simulink model "Boeing787_OldMission_ElectricalThermalHydraulicFuelECS"  (R2013a)
settings: Solver=ode23tb  SolverMode=SingleTasking  StartTime=0.0  StopTime=346  RelTol=1e-3
InitFcn:
  | load('SampleOutput.mat')
  | 
  | load('SampleFuelBurn.mat')
undefined symbols (not defined in the file or in its folder): ailerons, AirProp, B_737, elevator, FuelBurn, HydProp, landing_gear, rudder, thrust_rev
libraries: PowerFlowLib x118, simulink x20
(part 24 of 26)

== system Boeing787_OldMission_ElectricalThermalHydraulicFuelECS/ECS/Right Pack1/Primary HX (air-air)/Thermal_resistance_KpW_cold ==
  Convective_HTC : Inport
  HX_parameters : Inport  Port=2
  Fin_parameters : Inport  Port=3
  Add : Sum
  Bus Selector : BusSelector  OutputSignals=N_f
  Bus Selector1 : BusSelector  OutputSignals=s_fin,l_fin,eta_fin,h_fin
  Calc_R_tot : Product  Inputs=**
  Calc_R_tot1 : Product  Inputs=*/
  Constant : Constant  Value=2
  Gain : Gain  Gain=2
  R1_Convection_to_plate/fin_base : Product  Inputs=////
  R1_convection_fin_or_plate_base_KpW : Display
  R5_Conv-conduction_through fin_projection : Product  Inputs=//////
  R5_convection_fin_projection_KpW : Display
  R_tot_K/W : Outport
  wires:
  HX_parameters/1 -> Bus Selector/1
  Fin_parameters/1 -> Bus Selector1/1
  Convective_HTC/1 -> R1_Convection_to_plate/fin_base/1, R5_Conv-conduction_through fin_projection/3  "HTC_Wpm2K"
  Bus Selector/1 -> R1_Convection_to_plate/fin_base/2, R5_Conv-conduction_through fin_projection/4  "<N_f>"
  Bus Selector1/1 -> R1_Convection_to_plate/fin_base/3  "<s_fin>"
  Bus Selector1/2 -> R1_Convection_to_plate/fin_base/4, R5_Conv-conduction_through fin_projection/6  "<l_fin>"
  R1_Convection_to_plate/fin_base/1 -> R1_convection_fin_or_plate_base_KpW/1, Calc_R_tot/1, Add/1
  Constant/1 -> R5_Conv-conduction_through fin_projection/1
  Bus Selector1/3 -> R5_Conv-conduction_through fin_projection/2  "<eta_fin>"
  Bus Selector1/4 -> R5_Conv-conduction_through fin_projection/5  "<h_fin>"
  R5_Conv-conduction_through fin_projection/1 -> R5_convection_fin_projection_KpW/1, Calc_R_tot/2, Gain/1
  Gain/1 -> Add/2
  Calc_R_tot/1 -> Calc_R_tot1/1  "R1R5"
  Add/1 -> Calc_R_tot1/2  "R1+2R5"
  Calc_R_tot1/1 -> R_tot_K/W/1  "Rtot"

== system Boeing787_OldMission_ElectricalThermalHydraulicFuelECS/ECS/Right Pack1/Primary HX (air-air)/Thermal_resistance_KpW_hot ==
  Convective_HTC : Inport
  HX_parameters : Inport  Port=2
  Fin_parameters : Inport  Port=3
  Add : Sum
  Bus Selector : BusSelector  OutputSignals=N_f
  Bus Selector1 : BusSelector  OutputSignals=s_fin,l_fin,eta_fin,h_fin
  Calc_R_tot : Product  Inputs=**
  Calc_R_tot1 : Product  Inputs=*/
  Constant : Constant  Value=2
  Gain : Gain  Gain=2
  R1_Convection_to_plate/fin_base : Product  Inputs=////
  R1_convection_fin_or_plate_base_KpW : Display
  R5_Conv-conduction_through fin_projection : Product  Inputs=//////
  R5_convection_fin_projection_KpW : Display
  R_tot_K/W : Outport
  wires:
  Calc_R_tot1/1 -> R_tot_K/W/1  "Rtot"
  Add/1 -> Calc_R_tot1/2  "R1+2R5"
  Calc_R_tot/1 -> Calc_R_tot1/1  "R1R5"
  Gain/1 -> Add/2
  R5_Conv-conduction_through fin_projection/1 -> Gain/1, Calc_R_tot/2, R5_convection_fin_projection_KpW/1
  Bus Selector1/4 -> R5_Conv-conduction_through fin_projection/5  "<h_fin>"
  Bus Selector1/3 -> R5_Conv-conduction_through fin_projection/2  "<eta_fin>"
  Constant/1 -> R5_Conv-conduction_through fin_projection/1
  R1_Convection_to_plate/fin_base/1 -> Add/1, Calc_R_tot/1, R1_convection_fin_or_plate_base_KpW/1
  Bus Selector1/2 -> R5_Conv-conduction_through fin_projection/6, R1_Convection_to_plate/fin_base/4  "<l_fin>"
  Bus Selector1/1 -> R1_Convection_to_plate/fin_base/3  "<s_fin>"
  Bus Selector/1 -> R5_Conv-conduction_through fin_projection/4, R1_Convection_to_plate/fin_base/2  "<N_f>"
  Convective_HTC/1 -> R5_Conv-conduction_through fin_projection/3, R1_Convection_to_plate/fin_base/1  "HTC_Wpm2K"
  Fin_parameters/1 -> Bus Selector1/1
  HX_parameters/1 -> Bus Selector/1

== system Boeing787_OldMission_ElectricalThermalHydraulicFuelECS/ECS/Right Pack1/Primary HX (air-air)/convective_HTC_Wm-2K-1_cold ==
  Colburn_J_factor : Inport
  Re : Inport  Port=2
  air_properties : Inport  Port=3
  hydraulic_diameter : Inport  Port=4
  Bus Selector : BusSelector  OutputSignals=Pr,K_air
  Constant : Constant  Value=1/3
  Divide : Product  Inputs=****/
  Math Function : Math  Operator=pow  SaturateOnIntegerOverflow=on
  Convective_HTC_Wm-2K-1 : Outport
  wires:
  air_properties/1 -> Bus Selector/1
  Colburn_J_factor/1 -> Divide/1
  Re/1 -> Divide/2
  Bus Selector/1 -> Math Function/1  "<Pr>"
  Constant/1 -> Math Function/2
  Math Function/1 -> Divide/3
  Bus Selector/2 -> Divide/4  "<K_air>"
  hydraulic_diameter/1 -> Divide/5
  Divide/1 -> Convective_HTC_Wm-2K-1/1

== system Boeing787_OldMission_ElectricalThermalHydraulicFuelECS/ECS/Right Pack1/Primary HX (air-air)/convective_HTC_Wm-2K-1_hot ==
  Colburn_J_factor : Inport
  Re : Inport  Port=2
  air_properties : Inport  Port=3
  hydraulic_diameter : Inport  Port=4
  Bus Selector : BusSelector  OutputSignals=Pr,K_air
  Constant : Constant  Value=1/3
  Divide : Product  Inputs=****/
  Math Function : Math  Operator=pow  SaturateOnIntegerOverflow=on
  Convective_HTC_Wm-2K-1 : Outport
  wires:
  Divide/1 -> Convective_HTC_Wm-2K-1/1
  hydraulic_diameter/1 -> Divide/5
  Bus Selector/2 -> Divide/4  "<K_air>"
  Math Function/1 -> Divide/3
  Constant/1 -> Math Function/2
  Bus Selector/1 -> Math Function/1  "<Pr>"
  Re/1 -> Divide/2
  Colburn_J_factor/1 -> Divide/1
  air_properties/1 -> Bus Selector/1

== system Boeing787_OldMission_ElectricalThermalHydraulicFuelECS/ECS/Right Pack1/Secondary HX (air-air)1/Air_properties_in_flows_hot_and_cold ==
  In_flow_bus_hot : Inport
  In_flow_bus_cold : Inport  Port=2
  Bus Creator : BusCreator  Inputs=5
  Bus Creator3 : BusCreator  Inputs=5
  air_properties_in_cold : Subsystem
  air_properties_in_hot : Subsystem
  air_properties_in_hot1 : Outport
  air_properties_in_cold1 : Outport  Port=2
  wires:
  air_properties_in_hot/4(K_air_Wm-1K-2) -> Bus Creator/4  "K_air"
  air_properties_in_cold/5(Pr) -> Bus Creator3/5  "Pr"
  air_properties_in_hot/5(Pr) -> Bus Creator/5  "Pr"
  In_flow_bus_cold/1 -> air_properties_in_cold/1(In_flow_bus_cold)
  In_flow_bus_hot/1 -> air_properties_in_hot/1(In_flow_bus_hot)
  Bus Creator/1 -> air_properties_in_hot1/1
  Bus Creator3/1 -> air_properties_in_cold1/1
  air_properties_in_hot/3(mu_air_Pa.s) -> Bus Creator/3  "mu_air"
  air_properties_in_hot/2(cp_air_Jkg-1K-1) -> Bus Creator/2  "cp_air"
  air_properties_in_hot/1(rho_air_kgm-3) -> Bus Creator/1  "rho_air"
  air_properties_in_cold/4(K_air_Wm-1K-2) -> Bus Creator3/4  "K_air"
  air_properties_in_cold/3(mu_air_Pa.s) -> Bus Creator3/3  "mu_air"
  air_properties_in_cold/2(cp_air_Jkg-1K-1) -> Bus Creator3/2  "cp_air"
  air_properties_in_cold/1(rho_air_kgm-3) -> Bus Creator3/1  "rho_air"

== system Boeing787_OldMission_ElectricalThermalHydraulicFuelECS/ECS/Right Pack1/Secondary HX (air-air)1/C_T_c_av ==
  In_flow_bus : Inport
  air_properties : Inport  Port=2
  Tot_thermal_resist : Inport  Port=3
  Add : Sum
  Bus Selector : BusSelector  OutputSignals=mdot_kgps
  Bus Selector1 : BusSelector  OutputSignals=cp_air
  Constant : Constant
  Divide : Product  Inputs=***
  Divide1 : Product  Inputs=*/
  Gain : Gain  Gain=2
  C_T_c_av : Outport
  wires:
  Divide1/1 -> C_T_c_av/1
  Add/1 -> Divide1/2
  Constant/1 -> Add/2
  Gain/1 -> Divide1/1, Add/1
  Divide/1 -> Gain/1
  Bus Selector1/1 -> Divide/3  "<cp_air>"
  Bus Selector/1 -> Divide/2  "<mdot_kgps>"
  Tot_thermal_resist/1 -> Divide/1  "R_tot_c"
  In_flow_bus/1 -> Bus Selector/1
  air_properties/1 -> Bus Selector1/1

== system Boeing787_OldMission_ElectricalThermalHydraulicFuelECS/ECS/Right Pack1/Secondary HX (air-air)1/C_T_c_i ==
  In_flow_bus : Inport
  air_properties : Inport  Port=2
  Tot_thermal_resist : Inport  Port=3
  HX_parameters : Inport  Port=4
  Add : Sum
  Bus Selector : BusSelector  OutputSignals=mdot_kgps
  Bus Selector1 : BusSelector  OutputSignals=cp_air
  Bus Selector2 : BusSelector  OutputSignals=m_cm,cp_hx
  Constant : Constant
  Divide : Product  Inputs=***
  Divide2 : Product  Inputs=**///
  Gain : Gain  Gain=2
  Gain1 : Gain  Gain=2
  C_T_c_i : Outport
  wires:
  In_flow_bus/1 -> Bus Selector/1
  air_properties/1 -> Bus Selector1/1
  Tot_thermal_resist/1 -> Divide/1  "R_tot"
  Bus Selector/1 -> Divide/2, Divide2/1  "<mdot_kgps>"
  Bus Selector1/1 -> Divide/3, Divide2/2  "<cp_air>"
  Divide/1 -> Gain/1
  Gain/1 -> Add/1
  Constant/1 -> Add/2
  HX_parameters/1 -> Bus Selector2/1
  Bus Selector2/1 -> Divide2/3  "<m_cm>"
  Bus Selector2/2 -> Divide2/4  "<cp_hx>"
  Add/1 -> Divide2/5
  Gain1/1 -> C_T_c_i/1
  Divide2/1 -> Gain1/1

== system Boeing787_OldMission_ElectricalThermalHydraulicFuelECS/ECS/Right Pack1/Secondary HX (air-air)1/C_T_h_av ==
  In_flow_bus : Inport
  air_properties : Inport  Port=2
  Tot_thermal_resist : Inport  Port=3
  Add : Sum
  Bus Selector : BusSelector  OutputSignals=mdot_kgps
  Bus Selector1 : BusSelector  OutputSignals=cp_air
  Constant : Constant
  Divide : Product  Inputs=***
  Divide1 : Product  Inputs=*/
  Gain : Gain  Gain=2
  C_T_h_av : Outport
  wires:
  Divide1/1 -> C_T_h_av/1
  Add/1 -> Divide1/2
  Constant/1 -> Add/2
  Gain/1 -> Divide1/1, Add/1
  Divide/1 -> Gain/1
  Bus Selector1/1 -> Divide/3  "<cp_air>"
  Bus Selector/1 -> Divide/2  "<mdot_kgps>"
  Tot_thermal_resist/1 -> Divide/1  "R_tot_h"
  In_flow_bus/1 -> Bus Selector/1
  air_properties/1 -> Bus Selector1/1

== system Boeing787_OldMission_ElectricalThermalHydraulicFuelECS/ECS/Right Pack1/Secondary HX (air-air)1/C_T_h_i ==
  In_flow_bus : Inport
  air_properties : Inport  Port=2
  Tot_thermal_resist : Inport  Port=3
  HX_parameters : Inport  Port=4
  Add : Sum
  Bus Selector : BusSelector  OutputSignals=mdot_kgps
  Bus Selector1 : BusSelector  OutputSignals=cp_air
  Bus Selector2 : BusSelector  OutputSignals=m_cm,cp_hx
  Constant : Constant
  Divide : Product  Inputs=***
  Divide2 : Product  Inputs=**///
  Gain : Gain  Gain=2
  Gain1 : Gain  Gain=2
  C_T_h_i : Outport
  wires:
  Gain1/1 -> C_T_h_i/1
  Add/1 -> Divide2/5
  Bus Selector2/2 -> Divide2/4  "<cp_hx>"
  Bus Selector2/1 -> Divide2/3  "<m_cm>"
  HX_parameters/1 -> Bus Selector2/1
  Constant/1 -> Add/2
  Gain/1 -> Add/1
  Divide/1 -> Gain/1
  Bus Selector1/1 -> Divide/3, Divide2/2  "<cp_air>"
  Bus Selector/1 -> Divide/2, Divide2/1  "<mdot_kgps>"
  Tot_thermal_resist/1 -> Divide/1  "R_tot_h"
  air_properties/1 -> Bus Selector1/1
  In_flow_bus/1 -> Bus Selector/1
  Divide2/1 -> Gain1/1

== system Boeing787_OldMission_ElectricalThermalHydraulicFuelECS/ECS/Right Pack1/Secondary HX (air-air)1/Calculating_T_c_av ==
  T_cm : Inport
  In_flow_bus : Inport  Port=2
  C_t_c_av : Inport  Port=3
  Add1 : Sum  Inputs=-+
  Add3 : Sum
  Bus Selector : BusSelector  OutputSignals=temp_C
  Divide1 : Product  Inputs=**
  T_c_av_degreC : Outport
  wires:
  T_cm/1 -> Add3/1, Add1/1  "T_cm"
  In_flow_bus/1 -> Bus Selector/1
  Bus Selector/1 -> Add1/2  "<temp_C>"
  C_t_c_av/1 -> Divide1/2
  Add1/1 -> Divide1/1  "T_c_i - T_cm"
  Divide1/1 -> Add3/2
  Add3/1 -> T_c_av_degreC/1

== system Boeing787_OldMission_ElectricalThermalHydraulicFuelECS/ECS/Right Pack1/Secondary HX (air-air)1/Calculating_T_h_av ==
  T_cm : Inport
  In_flow_bus : Inport  Port=2
  C_t_h_av : Inport  Port=3
  Add1 : Sum  Inputs=-+
  Add3 : Sum
  Bus Selector : BusSelector  OutputSignals=temp_C
  Divide1 : Product  Inputs=**
  T_h_av_degreC : Outport
  wires:
  Add1/1 -> Divide1/1  "T_h_i - T_cm"
  C_t_h_av/1 -> Divide1/2
  Bus Selector/1 -> Add1/2  "<temp_C>"
  In_flow_bus/1 -> Bus Selector/1
  T_cm/1 -> Add1/1, Add3/1  "T_cm"
  Add3/1 -> T_h_av_degreC/1
  Divide1/1 -> Add3/2

== system Boeing787_OldMission_ElectricalThermalHydraulicFuelECS/ECS/Right Pack1/Secondary HX (air-air)1/Calculating_core_mass_temp ==
  note: dTcm/dt
  note: Tcm
  C_T_h_i : Inport
  C_T_c_i : Inport  Port=2
  C_t_cm : Inport  Port=3
  In_flow_bus_hot : Inport  Port=4
  In_flow_bus_cold : Inport  Port=5
  Add : Sum  Inputs=++-
  Bus Selector : BusSelector  OutputSignals=temp_C
  Bus Selector1 : BusSelector  OutputSignals=temp_C
  Divide : Product  Inputs=**
  Divide1 : Product  Inputs=**
  Divide2 : Product  Inputs=**
  Integrator : Integrator  InitialCondition=T_cm_0
  Core_mass_temp_C : Outport
  wires:
  Divide1/1 -> Add/3
  C_t_cm/1 -> Divide1/2
  Integrator/1 -> Core_mass_temp_C/1, Divide1/1
  Add/1 -> Integrator/1
  Divide2/1 -> Add/2
  Divide/1 -> Add/1
  Bus Selector1/1 -> Divide2/2  "<temp_C>"
  C_T_c_i/1 -> Divide2/1
  Bus Selector/1 -> Divide/2  "<temp_C>"
  C_T_h_i/1 -> Divide/1
  In_flow_bus_cold/1 -> Bus Selector1/1
  In_flow_bus_hot/1 -> Bus Selector/1

== system Boeing787_OldMission_ElectricalThermalHydraulicFuelECS/ECS/Right Pack1/Secondary HX (air-air)1/Colburn_J_factor_cold ==
  Fin_prameter_ratios : Inport
  Re : Inport  Port=2
  Add : Sum
  Bus Selector : BusSelector  OutputSignals=alpha_fin,delta_fin,gamma_fin
  Constant : Constant  Value=-0.5403
  Constant1 : Constant  Value=-0.1541
  Constant2 : Constant  Value=0.1499
  Constant3 : Constant  Value=-0.0678
  Constant4 : Constant  Value=1.34
  Constant5 : Constant  Value=0.504
  Constant6 : Constant  Value=0.456
  Constant7 : Constant  Value=-1.055
  Constant8 : Constant
  Constant9 : Constant  Value=0.1
  Divide : Product  Inputs=****
  Divide1 : Product  Inputs=****
  Divide2 : Product  Inputs=**
  Gain : Gain  Gain=0.6522
  Gain1 : Gain  Gain=5.269*10^(-5)
  Re1 : Math  Operator=pow  SaturateOnIntegerOverflow=on
  Re2 : Math  Operator=pow  SaturateOnIntegerOverflow=on
  alpha_fin : Math  Operator=pow  SaturateOnIntegerOverflow=on
  alpha_fin1 : Math  Operator=pow  SaturateOnIntegerOverflow=on
  delta_fin : Math  Operator=pow  SaturateOnIntegerOverflow=on
  delta_fin1 : Math  Operator=pow  SaturateOnIntegerOverflow=on
  gamma_fin : Math  Operator=pow  SaturateOnIntegerOverflow=on
  gamma_fin1 : Math  Operator=pow  SaturateOnIntegerOverflow=on
  gamma_fin2 : Math  Operator=pow  SaturateOnIntegerOverflow=on
  Colburn_J_factor : Outport
  wires:
  Divide2/1 -> Colburn_J_factor/1
  Gain/1 -> Divide2/1
  gamma_fin2/1 -> Divide2/2
  Constant9/1 -> gamma_fin2/2
  Add/1 -> gamma_fin2/1
  Gain1/1 -> Add/1
  Constant8/1 -> Add/2
  Divide1/1 -> Gain1/1
  gamma_fin1/1 -> Divide1/4
  delta_fin1/1 -> Divide1/3
  alpha_fin1/1 -> Divide1/2
  Re2/1 -> Divide1/1
  Divide/1 -> Gain/1
  gamma_fin/1 -> Divide/4
  delta_fin/1 -> Divide/3
  alpha_fin/1 -> Divide/2
  Re1/1 -> Divide/1
  Bus Selector/3 -> gamma_fin1/1, gamma_fin/1  "<gamma_fin>"
  Bus Selector/2 -> delta_fin1/1, delta_fin/1  "<delta_fin>"
  Bus Selector/1 -> alpha_fin1/1, alpha_fin/1  "<alpha_fin>"
  Re/1 -> Re2/1, Re1/1
  Constant7/1 -> gamma_fin1/2
  Constant6/1 -> delta_fin1/2
  Constant5/1 -> alpha_fin1/2
  Constant4/1 -> Re2/2
  Constant3/1 -> gamma_fin/2
  Constant2/1 -> delta_fin/2
  Constant1/1 -> alpha_fin/2
  Constant/1 -> Re1/2
  Fin_prameter_ratios/1 -> Bus Selector/1

== system Boeing787_OldMission_ElectricalThermalHydraulicFuelECS/ECS/Right Pack1/Secondary HX (air-air)1/Colburn_J_factor_hot ==
  Fin_prameter_ratios : Inport
  Re : Inport  Port=2
  Add : Sum
  Bus Selector : BusSelector  OutputSignals=alpha_fin,delta_fin,gamma_fin
  Constant : Constant  Value=-0.5403
  Constant1 : Constant  Value=-0.1541
  Constant2 : Constant  Value=0.1499
  Constant3 : Constant  Value=-0.0678
  Constant4 : Constant  Value=1.34
  Constant5 : Constant  Value=0.504
  Constant6 : Constant  Value=0.456
  Constant7 : Constant  Value=-1.055
  Constant8 : Constant
  Constant9 : Constant  Value=0.1
  Divide : Product  Inputs=****
  Divide1 : Product  Inputs=****
  Divide2 : Product  Inputs=**
  Gain : Gain  Gain=0.6522
  Gain1 : Gain  Gain=5.269*10^(-5)
  Re1 : Math  Operator=pow  SaturateOnIntegerOverflow=on
  Re2 : Math  Operator=pow  SaturateOnIntegerOverflow=on
  alpha_fin : Math  Operator=pow  SaturateOnIntegerOverflow=on
  alpha_fin1 : Math  Operator=pow  SaturateOnIntegerOverflow=on
  delta_fin : Math  Operator=pow  SaturateOnIntegerOverflow=on
  delta_fin1 : Math  Operator=pow  SaturateOnIntegerOverflow=on
  gamma_fin : Math  Operator=pow  SaturateOnIntegerOverflow=on
  gamma_fin1 : Math  Operator=pow  SaturateOnIntegerOverflow=on
  gamma_fin2 : Math  Operator=pow  SaturateOnIntegerOverflow=on
  Colburn_J_factor : Outport
  wires:
  Fin_prameter_ratios/1 -> Bus Selector/1
  Constant/1 -> Re1/2
  Constant1/1 -> alpha_fin/2
  Constant2/1 -> delta_fin/2
  Constant3/1 -> gamma_fin/2
  Constant4/1 -> Re2/2
  Constant5/1 -> alpha_fin1/2
  Constant6/1 -> delta_fin1/2
  Constant7/1 -> gamma_fin1/2
  Re/1 -> Re1/1, Re2/1
  Bus Selector/1 -> alpha_fin/1, alpha_fin1/1  "<alpha_fin>"
  Bus Selector/2 -> delta_fin/1, delta_fin1/1  "<delta_fin>"
  Bus Selector/3 -> gamma_fin/1, gamma_fin1/1  "<gamma_fin>"
  Re1/1 -> Divide/1
  alpha_fin/1 -> Divide/2
  delta_fin/1 -> Divide/3
  gamma_fin/1 -> Divide/4
  Divide/1 -> Gain/1
  Re2/1 -> Divide1/1
  alpha_fin1/1 -> Divide1/2
  delta_fin1/1 -> Divide1/3
  gamma_fin1/1 -> Divide1/4
  Divide1/1 -> Gain1/1
  Constant8/1 -> Add/2
  Gain1/1 -> Add/1
  Add/1 -> gamma_fin2/1
  Constant9/1 -> gamma_fin2/2
  gamma_fin2/1 -> Divide2/2
  Gain/1 -> Divide2/1
  Divide2/1 -> Colburn_J_factor/1

== system Boeing787_OldMission_ElectricalThermalHydraulicFuelECS/ECS/Right Pack1/Secondary HX (air-air)1/Friction_factor_cold ==
  Fin_prameter_ratios : Inport
  Re : Inport  Port=2
  Add : Sum
  Bus Selector : BusSelector  OutputSignals=alpha_fin,delta_fin,gamma_fin
  Constant : Constant  Value=-0.7422
  Constant1 : Constant  Value=-0.1856
  Constant2 : Constant  Value=0.3053
  Constant3 : Constant  Value=-0.2659
  Constant4 : Constant  Value=4.429
  Constant5 : Constant  Value=0.92
  Constant6 : Constant  Value=3.767
  Constant7 : Constant  Value=0.236
  Constant8 : Constant
  Constant9 : Constant  Value=0.1
  Divide : Product  Inputs=****
  Divide1 : Product  Inputs=****
  Divide2 : Product  Inputs=**
  Gain : Gain  Gain=9.6243
  Gain1 : Gain  Gain=7.669*10^(-8)
  Re1 : Math  Operator=pow  SaturateOnIntegerOverflow=on
  Re2 : Math  Operator=pow  SaturateOnIntegerOverflow=on
  alpha_fin : Math  Operator=pow  SaturateOnIntegerOverflow=on
  alpha_fin1 : Math  Operator=pow  SaturateOnIntegerOverflow=on
  delta_fin : Math  Operator=pow  SaturateOnIntegerOverflow=on
  delta_fin1 : Math  Operator=pow  SaturateOnIntegerOverflow=on
  gamma_fin : Math  Operator=pow  SaturateOnIntegerOverflow=on
  gamma_fin1 : Math  Operator=pow  SaturateOnIntegerOverflow=on
  gamma_fin2 : Math  Operator=pow  SaturateOnIntegerOverflow=on
  Friction_factor : Outport
  wires:
  Fin_prameter_ratios/1 -> Bus Selector/1
  Constant/1 -> Re1/2
  Constant1/1 -> alpha_fin/2
  Constant2/1 -> delta_fin/2
  Constant3/1 -> gamma_fin/2
  Constant4/1 -> Re2/2
  Constant5/1 -> alpha_fin1/2
  Constant6/1 -> delta_fin1/2
  Constant7/1 -> gamma_fin1/2
  Re/1 -> Re1/1, Re2/1
  Bus Selector/1 -> alpha_fin/1, alpha_fin1/1  "<alpha_fin>"
  Bus Selector/2 -> delta_fin/1, delta_fin1/1  "<delta_fin>"
  Bus Selector/3 -> gamma_fin/1, gamma_fin1/1  "<gamma_fin>"
  Re1/1 -> Divide/1
  alpha_fin/1 -> Divide/2
  delta_fin/1 -> Divide/3
  gamma_fin/1 -> Divide/4
  Divide/1 -> Gain/1
  Re2/1 -> Divide1/1
  alpha_fin1/1 -> Divide1/2
  delta_fin1/1 -> Divide1/3
  gamma_fin1/1 -> Divide1/4
  Divide1/1 -> Gain1/1
  Constant8/1 -> Add/2
  Gain1/1 -> Add/1
  Add/1 -> gamma_fin2/1
  Constant9/1 -> gamma_fin2/2
  gamma_fin2/1 -> Divide2/2
  Gain/1 -> Divide2/1
  Divide2/1 -> Friction_factor/1

== system Boeing787_OldMission_ElectricalThermalHydraulicFuelECS/ECS/Right Pack1/Secondary HX (air-air)1/Friction_factor_hot ==
  Fin_prameter_ratios : Inport
  Re : Inport  Port=2
  Add : Sum
  Bus Selector : BusSelector  OutputSignals=alpha_fin,delta_fin,gamma_fin
  Constant : Constant  Value=-0.7422
  Constant1 : Constant  Value=-0.1856
  Constant2 : Constant  Value=0.3053
  Constant3 : Constant  Value=-0.2659
  Constant4 : Constant  Value=4.429
  Constant5 : Constant  Value=0.92
  Constant6 : Constant  Value=3.767
  Constant7 : Constant  Value=0.236
  Constant8 : Constant
  Constant9 : Constant  Value=0.1
  Divide : Product  Inputs=****
  Divide1 : Product  Inputs=****
  Divide2 : Product  Inputs=**
  Gain : Gain  Gain=9.6243
  Gain1 : Gain  Gain=7.669*10^(-8)
  Re1 : Math  Operator=pow  SaturateOnIntegerOverflow=on
  Re2 : Math  Operator=pow  SaturateOnIntegerOverflow=on
  alpha_fin : Math  Operator=pow  SaturateOnIntegerOverflow=on
  alpha_fin1 : Math  Operator=pow  SaturateOnIntegerOverflow=on
  delta_fin : Math  Operator=pow  SaturateOnIntegerOverflow=on
  delta_fin1 : Math  Operator=pow  SaturateOnIntegerOverflow=on
  gamma_fin : Math  Operator=pow  SaturateOnIntegerOverflow=on
  gamma_fin1 : Math  Operator=pow  SaturateOnIntegerOverflow=on
  gamma_fin2 : Math  Operator=pow  SaturateOnIntegerOverflow=on
  Friction_factor : Outport
  wires:
  Divide2/1 -> Friction_factor/1
  Gain/1 -> Divide2/1
  gamma_fin2/1 -> Divide2/2
  Constant9/1 -> gamma_fin2/2
  Add/1 -> gamma_fin2/1
  Gain1/1 -> Add/1
  Constant8/1 -> Add/2
  Divide1/1 -> Gain1/1
  gamma_fin1/1 -> Divide1/4
  delta_fin1/1 -> Divide1/3
  alpha_fin1/1 -> Divide1/2
  Re2/1 -> Divide1/1
  Divide/1 -> Gain/1
  gamma_fin/1 -> Divide/4
  delta_fin/1 -> Divide/3
  alpha_fin/1 -> Divide/2
  Re1/1 -> Divide/1
  Bus Selector/3 -> gamma_fin1/1, gamma_fin/1  "<gamma_fin>"
  Bus Selector/2 -> delta_fin1/1, delta_fin/1  "<delta_fin>"
  Bus Selector/1 -> alpha_fin1/1, alpha_fin/1  "<alpha_fin>"
  Re/1 -> Re2/1, Re1/1
  Constant7/1 -> gamma_fin1/2
  Constant6/1 -> delta_fin1/2
  Constant5/1 -> alpha_fin1/2
  Constant4/1 -> Re2/2
  Constant3/1 -> gamma_fin/2
  Constant2/1 -> delta_fin/2
  Constant1/1 -> alpha_fin/2
  Constant/1 -> Re1/2
  Fin_prameter_ratios/1 -> Bus Selector/1

== system Boeing787_OldMission_ElectricalThermalHydraulicFuelECS/ECS/Right Pack1/Secondary HX (air-air)1/HX_and_Fin_paramters ==
  Bus Creator1 : BusCreator  Inputs=6
  Bus Creator2 : BusCreator  Inputs=6
  Bus Creator3 : BusCreator  Inputs=3
  Fin_parameters : Subsystem
  HX_parameters : Subsystem
  Other_HX_parameters2 : Subsystem
  alpha : Product  Inputs=*/
  delta : Product  Inputs=*/
  gamma : Product  Inputs=*/
  HX_parameters2 : Outport
  Fin_parameters1 : Outport  Port=2
  Fin_parameters_ratios : Outport  Port=3
  wires:
  [Other_HX_parameters] -> HX_parameters/1(Other_HX_parameters)
  Other_HX_parameters2/1(Out1) -> [Other_HX_parameters]
  Bus Creator3/1 -> Fin_parameters_ratios/1
  gamma/1 -> Bus Creator3/3  "gamma_fin"
  delta/1 -> Bus Creator3/2  "delta_fin"
  alpha/1 -> Bus Creator3/1  "alpha_fin"
  Bus Creator1/1 -> HX_parameters2/1
  Bus Creator2/1 -> HX_parameters/2(Fin_parameters), Fin_parameters1/1
  HX_parameters/1(tot_free_flow_area_m^2) -> Bus Creator1/1  "A"
  Fin_parameters/3(Fin_free_flow_width_m) -> Bus Creator2/3, alpha/1, gamma/2  "s_fin"
  Fin_parameters/6(Fin_eff) -> Bus Creator2/6  "eta_fin"
  Fin_parameters/5(K_fin_Wm-1K-1) -> Bus Creator2/5  "K_n"
  Fin_parameters/4(Fin_free_flow_height_m) -> Bus Creator2/4, alpha/2  "h_fin"
  Fin_parameters/2(Fin_thickness_m) -> gamma/1, Bus Creator2/2, delta/1  "t_fin"
  Fin_parameters/1(Fin_length_m) -> Bus Creator2/1, delta/2  "l_fin"
  HX_parameters/6(m_hx_kg) -> Bus Creator1/6  "m_cm"
  HX_parameters/5(cp_hx_Jkg-1K-1) -> Bus Creator1/5  "cp_hx"
  HX_parameters/4(K_hx_Wm-1K-1) -> Bus Creator1/4  "K_p"
  HX_parameters/3(tot_no_of_fins_per_HX_per_flow) -> Bus Creator1/3  "N_f"
  HX_parameters/2(tot_length_in_direc_of_flow_m) -> Bus Creator1/2  "L_hx"

== system Boeing787_OldMission_ElectricalThermalHydraulicFuelECS/ECS/Right Pack1/Secondary HX (air-air)1/Heat_load_cold_side ==
  In_flow_bus : Inport
  air_properties : Inport  Port=2
  temp_out_degreeC : Inport  Port=3
  Bus Selector : BusSelector  OutputSignals=temp_C,mdot_kgps
  Bus Selector1 : BusSelector  OutputSignals=cp_air
  Product : Product  Inputs=3  RndMeth=Zero
  temp_diff : Sum  Inputs=-+
  Heat_rate_Watt : Outport
  wires:
  In_flow_bus/1 -> Bus Selector/1
  air_properties/1 -> Bus Selector1/1
  Bus Selector/1 -> temp_diff/1  "<temp_C>"
  temp_out_degreeC/1 -> temp_diff/2
  Bus Selector/2 -> Product/1  "<mdot_kgps>"
  Bus Selector1/1 -> Product/2  "<cp_air>"
  temp_diff/1 -> Product/3
  Product/1 -> Heat_rate_Watt/1

== system Boeing787_OldMission_ElectricalThermalHydraulicFuelECS/ECS/Right Pack1/Secondary HX (air-air)1/Heat_load_hot_side ==
  In_flow_bus : Inport
  air_properties : Inport  Port=2
  temp_out_degreeC : Inport  Port=3
  Bus Selector : BusSelector  OutputSignals=temp_C,mdot_kgps
  Bus Selector1 : BusSelector  OutputSignals=cp_air
  Product : Product  Inputs=3  RndMeth=Zero
  temp_diff : Sum  Inputs=+-
  Heat_rate_Watt : Outport
  wires:
  Product/1 -> Heat_rate_Watt/1
  temp_diff/1 -> Product/3
  Bus Selector1/1 -> Product/2  "<cp_air>"
  Bus Selector/2 -> Product/1  "<mdot_kgps>"
  temp_out_degreeC/1 -> temp_diff/2
  Bus Selector/1 -> temp_diff/1  "<temp_C>"
  air_properties/1 -> Bus Selector1/1
  In_flow_bus/1 -> Bus Selector/1

== system Boeing787_OldMission_ElectricalThermalHydraulicFuelECS/ECS/Right Pack1/Secondary HX (air-air)1/Hydraulic_diam_m ==
  Fin_parameters : Inport
  Add : Sum  Inputs=+++
  Add1 : Sum
  Bus Selector1 : BusSelector  OutputSignals=l_fin,t_fin,s_fin,h_fin,K_n,eta_fin
  Gain : Gain  Gain=4
  Gain1 : Gain  Gain=2
  Terminator : Terminator
  Terminator1 : Terminator
  hl : Product  Inputs=**
  shl : Product  Inputs=***
  sl : Product  Inputs=**
  th : Product  Inputs=**
  ts : Product  Inputs=**
  ts1 : Product  Inputs=*/
  Out1 : Outport
  wires:
  ts1/1 -> Out1/1
  Add1/1 -> ts1/2
  Gain/1 -> ts1/1
  ts/1 -> Add1/2
  Gain1/1 -> Add1/1
  Add/1 -> Gain1/1
  th/1 -> Add/3
  hl/1 -> Add/2
  sl/1 -> Add/1
  Bus Selector1/2 -> th/1, ts/1  "<t_fin>"
  shl/1 -> Gain/1
  Bus Selector1/1 -> hl/2, sl/2, shl/3  "<l_fin>"
  Bus Selector1/4 -> th/2, shl/2, hl/1  "<h_fin>"
  Bus Selector1/3 -> ts/2, sl/1, shl/1  "<s_fin>"
  Fin_parameters/1 -> Bus Selector1/1
  Bus Selector1/5 -> Terminator/1  "<K_n>"
  Bus Selector1/6 -> Terminator1/1  "<eta_fin>"

== system Boeing787_OldMission_ElectricalThermalHydraulicFuelECS/ECS/Right Pack1/Secondary HX (air-air)1/Pressure_drop_cold ==
  Friction_factor : Inport
  HX_parameters : Inport  Port=2
  air_properties : Inport  Port=3
  air_velocity : Inport  Port=4
  D_hydraulic : Inport  Port=5
  In_flow_bus : Inport  Port=6
  Add : Sum  Inputs=-+
  Bus Selector : BusSelector  OutputSignals=L_hx
  Bus Selector1 : BusSelector  OutputSignals=rho_air
  Bus Selector2 : BusSelector  OutputSignals=press_Pa
  Constant : Constant  Value=2
  Divide3 : Product  Inputs=****/
  Gain2 : Gain  Gain=2
  Math Function : Math  Operator=pow  SaturateOnIntegerOverflow=on
  pres_drop_Pa : Outport
  pres_Pa : Outport  Port=2
  wires:
  Friction_factor/1 -> Divide3/1
  HX_parameters/1 -> Bus Selector/1
  Bus Selector/1 -> Divide3/2  "<L_hx>"
  air_properties/1 -> Bus Selector1/1
  Bus Selector1/1 -> Divide3/3  "<rho_air>"
  air_velocity/1 -> Math Function/1
  Constant/1 -> Math Function/2
  Math Function/1 -> Divide3/4
  D_hydraulic/1 -> Divide3/5
  Divide3/1 -> Gain2/1
  Gain2/1 -> pres_drop_Pa/1, Add/1  "pres_drop_Pa"
  In_flow_bus/1 -> Bus Selector2/1
  Bus Selector2/1 -> Add/2  "<press_Pa>"
  Add/1 -> pres_Pa/1

== system Boeing787_OldMission_ElectricalThermalHydraulicFuelECS/ECS/Right Pack1/Secondary HX (air-air)1/Pressure_drop_hot ==
  Friction_factor : Inport
  HX_parameters : Inport  Port=2
  air_properties : Inport  Port=3
  air_velocity : Inport  Port=4
  D_hydraulic : Inport  Port=5
  In_flow_bus : Inport  Port=6
  Add : Sum  Inputs=-+
  Bus Selector : BusSelector  OutputSignals=L_hx
  Bus Selector1 : BusSelector  OutputSignals=rho_air
  Bus Selector2 : BusSelector  OutputSignals=pres_Pa
  Constant : Constant  Value=2
  Divide3 : Product  Inputs=****/
  Gain2 : Gain  Gain=2
  Math Function : Math  Operator=pow  SaturateOnIntegerOverflow=on
  pres_drop_Pa : Outport
  pres_Pa : Outport  Port=2
  wires:
  Add/1 -> pres_Pa/1
  Bus Selector2/1 -> Add/2  "<pres_Pa>"
  In_flow_bus/1 -> Bus Selector2/1
  Gain2/1 -> Add/1, pres_drop_Pa/1  "pres_drop_Pa"
  Divide3/1 -> Gain2/1
  D_hydraulic/1 -> Divide3/5
  Math Function/1 -> Divide3/4
  Constant/1 -> Math Function/2
  air_velocity/1 -> Math Function/1
  Bus Selector1/1 -> Divide3/3  "<rho_air>"
  air_properties/1 -> Bus Selector1/1
  Bus Selector/1 -> Divide3/2  "<L_hx>"
  HX_parameters/1 -> Bus Selector/1
  Friction_factor/1 -> Divide3/1

== system Boeing787_OldMission_ElectricalThermalHydraulicFuelECS/ECS/Right Pack1/Secondary HX (air-air)1/Re_number_in_cold ==
  In_flow_bus : Inport
  air_properties : Inport  Port=2
  Hydraulic_diam : Inport  Port=3
  HX_paramters : Inport  Port=4
  Bus Selector : BusSelector  OutputSignals=mdot_kgps
  Bus Selector1 : BusSelector  OutputSignals=rho_air,mu_air
  Bus Selector2 : BusSelector  OutputSignals=A
  Re_number_claculation : Product  Inputs=***/
  Velocity_calculation : Product  Inputs=*//
  Re_number : Outport
  velo_air_ms-1 : Outport  Port=2
  wires:
  air_properties/1 -> Bus Selector1/1
  In_flow_bus/1 -> Bus Selector/1
  HX_paramters/1 -> Bus Selector2/1
  Bus Selector/1 -> Velocity_calculation/1  "<mdot_kgps>"
  Bus Selector1/1 -> Velocity_calculation/2, Re_number_claculation/1  "<rho_air>"
  Bus Selector2/1 -> Velocity_calculation/3  "<A>"
  Velocity_calculation/1 -> velo_air_ms-1/1, Re_number_claculation/2  "Velo_air_ms-1"
  Hydraulic_diam/1 -> Re_number_claculation/3
  Bus Selector1/2 -> Re_number_claculation/4  "<mu_air>"
  Re_number_claculation/1 -> Re_number/1  "Re_number"

== system Boeing787_OldMission_ElectricalThermalHydraulicFuelECS/ECS/Right Pack1/Secondary HX (air-air)1/Re_number_in_hot ==
  In_flow_bus : Inport
  air_properties : Inport  Port=2
  Hydraulic_diam : Inport  Port=3
  HX_paramters : Inport  Port=4
  Bus Selector : BusSelector  OutputSignals=mdot_kgps
  Bus Selector1 : BusSelector  OutputSignals=rho_air,mu_air
  Bus Selector2 : BusSelector  OutputSignals=A
  Re_number_claculation : Product  Inputs=***/
  Velocity_calculation : Product  Inputs=*//
  Re_number : Outport
  velo_air_ms-1 : Outport  Port=2
  wires:
  Re_number_claculation/1 -> Re_number/1  "Re_number"
  Bus Selector1/2 -> Re_number_claculation/4  "<mu_air>"
  Hydraulic_diam/1 -> Re_number_claculation/3
  Velocity_calculation/1 -> velo_air_ms-1/1, Re_number_claculation/2  "Velo_air_ms-1"
  Bus Selector2/1 -> Velocity_calculation/3  "<A>"
  Bus Selector1/1 -> Re_number_claculation/1, Velocity_calculation/2  "<rho_air>"
  Bus Selector/1 -> Velocity_calculation/1  "<mdot_kgps>"
  HX_paramters/1 -> Bus Selector2/1
  In_flow_bus/1 -> Bus Selector/1
  air_properties/1 -> Bus Selector1/1

== system Boeing787_OldMission_ElectricalThermalHydraulicFuelECS/ECS/Right Pack1/Secondary HX (air-air)1/Thermal_resistance_KpW_cold ==
  Convective_HTC : Inport
  HX_parameters : Inport  Port=2
  Fin_parameters : Inport  Port=3
  Add : Sum
  Bus Selector : BusSelector  OutputSignals=N_f
  Bus Selector1 : BusSelector  OutputSignals=s_fin,l_fin,eta_fin,h_fin
  Calc_R_tot : Product  Inputs=**
  Calc_R_tot1 : Product  Inputs=*/
  Constant : Constant  Value=2
  Gain : Gain  Gain=2
  R1_Convection_to_plate/fin_base : Product  Inputs=////
  R1_convection_fin_or_plate_base_KpW : Display
  R5_Conv-conduction_through fin_projection : Product  Inputs=//////
  R5_convection_fin_projection_KpW : Display
  R_tot_K/W : Outport
  wires:
  HX_parameters/1 -> Bus Selector/1
  Fin_parameters/1 -> Bus Selector1/1
  Convective_HTC/1 -> R1_Convection_to_plate/fin_base/1, R5_Conv-conduction_through fin_projection/3  "HTC_Wpm2K"
  Bus Selector/1 -> R1_Convection_to_plate/fin_base/2, R5_Conv-conduction_through fin_projection/4  "<N_f>"
  Bus Selector1/1 -> R1_Convection_to_plate/fin_base/3  "<s_fin>"
  Bus Selector1/2 -> R1_Convection_to_plate/fin_base/4, R5_Conv-conduction_through fin_projection/6  "<l_fin>"
  R1_Convection_to_plate/fin_base/1 -> R1_convection_fin_or_plate_base_KpW/1, Calc_R_tot/1, Add/1
  Constant/1 -> R5_Conv-conduction_through fin_projection/1
  Bus Selector1/3 -> R5_Conv-conduction_through fin_projection/2  "<eta_fin>"
  Bus Selector1/4 -> R5_Conv-conduction_through fin_projection/5  "<h_fin>"
  R5_Conv-conduction_through fin_projection/1 -> R5_convection_fin_projection_KpW/1, Calc_R_tot/2, Gain/1
  Gain/1 -> Add/2
  Calc_R_tot/1 -> Calc_R_tot1/1  "R1R5"
  Add/1 -> Calc_R_tot1/2  "R1+2R5"
  Calc_R_tot1/1 -> R_tot_K/W/1  "Rtot"

== system Boeing787_OldMission_ElectricalThermalHydraulicFuelECS/ECS/Right Pack1/Secondary HX (air-air)1/Thermal_resistance_KpW_hot ==
  Convective_HTC : Inport
  HX_parameters : Inport  Port=2
  Fin_parameters : Inport  Port=3
  Add : Sum
  Bus Selector : BusSelector  OutputSignals=N_f
  Bus Selector1 : BusSelector  OutputSignals=s_fin,l_fin,eta_fin,h_fin
  Calc_R_tot : Product  Inputs=**
  Calc_R_tot1 : Product  Inputs=*/
  Constant : Constant  Value=2
  Gain : Gain  Gain=2
  R1_Convection_to_plate/fin_base : Product  Inputs=////
  R1_convection_fin_or_plate_base_KpW : Display
  R5_Conv-conduction_through fin_projection : Product  Inputs=//////
  R5_convection_fin_projection_KpW : Display
  R_tot_K/W : Outport
  wires:
  Calc_R_tot1/1 -> R_tot_K/W/1  "Rtot"
  Add/1 -> Calc_R_tot1/2  "R1+2R5"
  Calc_R_tot/1 -> Calc_R_tot1/1  "R1R5"
  Gain/1 -> Add/2
  R5_Conv-conduction_through fin_projection/1 -> Gain/1, Calc_R_tot/2, R5_convection_fin_projection_KpW/1
  Bus Selector1/4 -> R5_Conv-conduction_through fin_projection/5  "<h_fin>"
  Bus Selector1/3 -> R5_Conv-conduction_through fin_projection/2  "<eta_fin>"
  Constant/1 -> R5_Conv-conduction_through fin_projection/1
  R1_Convection_to_plate/fin_base/1 -> Add/1, Calc_R_tot/1, R1_convection_fin_or_plate_base_KpW/1
  Bus Selector1/2 -> R5_Conv-conduction_through fin_projection/6, R1_Convection_to_plate/fin_base/4  "<l_fin>"
  Bus Selector1/1 -> R1_Convection_to_plate/fin_base/3  "<s_fin>"
  Bus Selector/1 -> R5_Conv-conduction_through fin_projection/4, R1_Convection_to_plate/fin_base/2  "<N_f>"
  Convective_HTC/1 -> R5_Conv-conduction_through fin_projection/3, R1_Convection_to_plate/fin_base/1  "HTC_Wpm2K"
  Fin_parameters/1 -> Bus Selector1/1
  HX_parameters/1 -> Bus Selector/1

== system Boeing787_OldMission_ElectricalThermalHydraulicFuelECS/ECS/Right Pack1/Secondary HX (air-air)1/convective_HTC_Wm-2K-1_cold ==
  Colburn_J_factor : Inport
  Re : Inport  Port=2
  air_properties : Inport  Port=3
  hydraulic_diameter : Inport  Port=4
  Bus Selector : BusSelector  OutputSignals=Pr,K_air
  Constant : Constant  Value=1/3
  Divide : Product  Inputs=****/
  Math Function : Math  Operator=pow  SaturateOnIntegerOverflow=on
  Convective_HTC_Wm-2K-1 : Outport
  wires:
  air_properties/1 -> Bus Selector/1
  Colburn_J_factor/1 -> Divide/1
  Re/1 -> Divide/2
  Bus Selector/1 -> Math Function/1  "<Pr>"
  Constant/1 -> Math Function/2
  Math Function/1 -> Divide/3
  Bus Selector/2 -> Divide/4  "<K_air>"
  hydraulic_diameter/1 -> Divide/5
  Divide/1 -> Convective_HTC_Wm-2K-1/1

== system Boeing787_OldMission_ElectricalThermalHydraulicFuelECS/ECS/Right Pack1/Secondary HX (air-air)1/convective_HTC_Wm-2K-1_hot ==
  Colburn_J_factor : Inport
  Re : Inport  Port=2
  air_properties : Inport  Port=3
  hydraulic_diameter : Inport  Port=4
  Bus Selector : BusSelector  OutputSignals=Pr,K_air
  Constant : Constant  Value=1/3
  Divide : Product  Inputs=****/
  Math Function : Math  Operator=pow  SaturateOnIntegerOverflow=on
  Convective_HTC_Wm-2K-1 : Outport
  wires:
  Divide/1 -> Convective_HTC_Wm-2K-1/1
  hydraulic_diameter/1 -> Divide/5
  Bus Selector/2 -> Divide/4  "<K_air>"
  Math Function/1 -> Divide/3
  Constant/1 -> Math Function/2
  Bus Selector/1 -> Math Function/1  "<Pr>"
  Re/1 -> Divide/2
  Colburn_J_factor/1 -> Divide/1
  air_properties/1 -> Bus Selector/1

== system Boeing787_OldMission_ElectricalThermalHydraulicFuelECS/Electrical/Enabled_AC_Loadloss/Enabled Subsystem/CURRENT BASED LOADS ==
  note: SPLITTING CURRENT IN BOTH D AND Q AXES
  Constant : Constant  Value=0
  Constant1 : Constant  Value=ILRMS
  Gain1 : Gain  Gain=sqrt(2)
  Mux : Mux  Inputs=3
  Idqo : Outport
  wires:
  Constant/1 -> Mux/3
  Mux/1 -> Idqo/1
  Gain1/1 -> Mux/2, Mux/1
  Constant1/1 -> Gain1/1

== system Boeing787_OldMission_ElectricalThermalHydraulicFuelECS/Electrical/Enabled_AC_Loadloss/Enabled Subsystem/IMPEDANCE BASED LOADS ==
  Vdq0 : Inport
  Constant1 : Constant  Value=R
  Constant2 : Constant  Value=X
  Constant3 : Constant  Value=R
  Constant4 : Constant  Value=X
  Demux : Demux  Outputs=3
  Fcn : Fcn  Expr=u(1)/(u(2)+0.1)
  Fcn1 : Fcn  Expr=u(1)/(u(2)+0.1)
  Math Function{,1..3} (4 alike) : Math  Operator=square  SaturateOnIntegerOverflow=on
  Mux : Mux  Inputs=3
  Mux1 : Mux  Inputs=2
  Mux2 : Mux  Inputs=2
  Product{1..2,5..6} (4 alike) : Product  Inputs=**  RndMeth=Zero
  Sum1 : Sum  Inputs=|++
  Sum2 : Sum  Inputs=|++
  Sum3 : Sum  Inputs=|+-
  Sum4 : Sum  Inputs=|++
  Idq0 : Outport
  wires:
  Fcn1/1 -> Mux/2
  Fcn/1 -> Mux/1
  Vdq0/1 -> Demux/1
  Constant1/1 -> Product1/1, Math Function/1
  Demux/1 -> Product1/2, Product6/2
  Product1/1 -> Sum1/1
  Demux/2 -> Product2/2, Product5/2
  Constant2/1 -> Product2/1, Math Function1/1
  Product2/1 -> Sum1/2
  Sum1/1 -> Mux1/1
  Math Function/1 -> Sum2/1
  Math Function1/1 -> Sum2/2
  Sum2/1 -> Mux1/2
  Constant3/1 -> Product5/1, Math Function2/1
  Product5/1 -> Sum3/1
  Constant4/1 -> Product6/1, Math Function3/1
  Product6/1 -> Sum3/2
  Math Function2/1 -> Sum4/1
  Math Function3/1 -> Sum4/2
  Sum3/1 -> Mux2/1
  Sum4/1 -> Mux2/2
  Mux1/1 -> Fcn/1
  Mux2/1 -> Fcn1/1
  Mux/1 -> Idq0/1

== system Boeing787_OldMission_ElectricalThermalHydraulicFuelECS/Electrical/Enabled_AC_Loadloss/Enabled Subsystem/POWER BASED LOADS ==
  Vdq0 : Inport
  Constant1 : Constant  Value=P
  Constant2 : Constant  Value=PF
  Constant3 : Constant  Value=P
  Constant5 : Constant
  Constant6 : Constant  Value=0
  Constant7 : Constant  Value=P
  Demux : Demux  Outputs=3
  Fcn : Fcn  Expr=u(1)/(u(2)+0.1)
  Fcn1 : Fcn  Expr=u(1)/(u(2)+0.1)
  Math Function{,1..3} (4 alike) : Math  Operator=square  SaturateOnIntegerOverflow=on
  Mux : Mux  Inputs=3
  Mux1 : Mux  Inputs=2
  Mux2 : Mux  Inputs=2
  Product1 : Product  Inputs=***  RndMeth=Zero
  Product2 : Product  Inputs=**  RndMeth=Zero
  Product3 : Product  Inputs=**  RndMeth=Zero
  Product5 : Product  Inputs=***  RndMeth=Zero
  Product6 : Product  Inputs=**  RndMeth=Zero
  Sum1 : Sum  Inputs=|++
  Sum2 : Sum  Inputs=|++
  Sum3 : Sum  Inputs=|+-
  Sum4 : Sum  Inputs=|++
  Trigonometric Function : Trigonometry  Operator=acos
  Trigonometric Function1 : Trigonometry  Operator=tan
  Idq0 : Outport
  loss : Outport  Port=2
  wires:
  Constant1/1 -> Product1/1, loss/1
  Constant6/1 -> Product5/3
  Constant5/1 -> Product1/3
  Mux/1 -> Idq0/1
  Mux2/1 -> Fcn1/1
  Mux1/1 -> Fcn/1
  Sum4/1 -> Mux2/2
  Sum3/1 -> Mux2/1
  Math Function3/1 -> Sum4/2
  Math Function2/1 -> Sum4/1
  Product6/1 -> Sum3/2
  Product3/1 -> Product6/1, Product2/1
  Product5/1 -> Sum3/1
  Constant3/1 -> Product5/1
  Sum2/1 -> Mux1/2
  Math Function1/1 -> Sum2/2
  Math Function/1 -> Sum2/1
  Sum1/1 -> Mux1/1
  Product2/1 -> Sum1/2
  Constant2/1 -> Trigonometric Function/1
  Demux/2 -> Math Function2/1, Product5/2, Math Function1/1, Product2/2
  Product1/1 -> Sum1/1
  Demux/1 -> Math Function3/1, Product6/2, Math Function/1, Product1/2
  Vdq0/1 -> Demux/1
  Fcn/1 -> Mux/1
  Fcn1/1 -> Mux/2
  Trigonometric Function/1 -> Trigonometric Function1/1
  Trigonometric Function1/1 -> Product3/1
  Constant7/1 -> Product3/2

== system Boeing787_OldMission_ElectricalThermalHydraulicFuelECS/Electrical/Enabled_AC_Loadloss/Enabled Subsystem1/CURRENT BASED LOADS ==
  note: SPLITTING CURRENT IN BOTH D AND Q AXES
  Iconst RMS : Inport
  Gain1 : Gain  Gain=sqrt(2)
  Mux : Mux  Inputs=3
  Idqo : Outport
  wires:
  Iconst RMS/1 -> Gain1/1
  Gain1/1 -> Mux/1, Mux/2
  Mux/1 -> Idqo/1

== system Boeing787_OldMission_ElectricalThermalHydraulicFuelECS/Electrical/Enabled_AC_Loadloss/Enabled Subsystem1/POWER BASED LOADS ==
  Vdq0 : Inport
  P : Inport  Port=2
  Q : Inport  Port=3
  Demux : Demux  Outputs=3
  Fcn : Fcn  Expr=u(1)/(u(2)+0.1)
  Fcn1 : Fcn  Expr=u(1)/(u(2)+0.1)
  Math Function{,1..3} (4 alike) : Math  Operator=square  SaturateOnIntegerOverflow=on
  Mux : Mux  Inputs=3
  Mux1 : Mux  Inputs=2
  Mux2 : Mux  Inputs=2
  Product{1..2,5..6} (4 alike) : Product  Inputs=**  RndMeth=Zero
  Sum1 : Sum  Inputs=|++
  Sum2 : Sum  Inputs=|++
  Sum3 : Sum  Inputs=|+-
  Sum4 : Sum  Inputs=|++
  Idq0 : Outport
  wires:
  Demux/1 -> Math Function/1, Product1/2, Product6/2, Math Function3/1
  Vdq0/1 -> Demux/1
  P/1 -> Product1/1, Product5/1
  Product1/1 -> Sum1/1
  Demux/2 -> Product2/2, Math Function1/1, Product5/2, Math Function2/1
  Q/1 -> Product2/1, Product6/1
  Product2/1 -> Sum1/2
  Sum1/1 -> Mux1/1
  Math Function/1 -> Sum2/1
  Math Function1/1 -> Sum2/2
  Sum2/1 -> Mux1/2
  Product5/1 -> Sum3/1
  Product6/1 -> Sum3/2
  Math Function2/1 -> Sum4/1
  Math Function3/1 -> Sum4/2
  Sum3/1 -> Mux2/1
  Sum4/1 -> Mux2/2
  Mux1/1 -> Fcn/1
  Mux2/1 -> Fcn1/1
  Mux/1 -> Idq0/1
  Fcn/1 -> Mux/1
  Fcn1/1 -> Mux/2

== system Boeing787_OldMission_ElectricalThermalHydraulicFuelECS/Electrical/Generation Unit Sync-Sync1/Generator/Dynamics ==
  Id : Inport
  Iq : Inport  Port=2
  Efd : Inport  Port=3
  Temp : Inport  Port=4
  Gain : Gain  Gain=Xd1 - Xls
  Gain1 : Gain  Gain=(Xd1 - Xd2)/(Xd1-Xls)^2
  Gain10 : Gain  Gain=Xq1 - Xls
  Gain11 : Gain  Gain=1/Tqo2
  Gain2 : Gain  Gain=Xd - Xd1
  Gain3 : Gain  Gain=1/Tdo1
  Gain4 : Gain  Gain=Xq1 - Xls
  Gain5 : Gain  Gain=(Xq1 - Xq2)/(Xq1 - Xls)^2
  Gain6 : Gain  Gain=Xq - Xq1
  Gain7 : Gain  Gain=1/Tqo1
  Gain8 : Gain  Gain=Xd1 - Xls
  Gain9 : Gain  Gain=1/Tdo2
  Integrator{,1..3} (4 alike) : Integrator
  Product{1..4} (4 alike) : Product
  Sum : Sum  Inputs=++-
  Sum1 : Sum  Inputs=+-
  Sum2 : Sum  Inputs=--+
  Sum3 : Sum  Inputs=+++
  Sum4 : Sum  Inputs=+-
  Sum5 : Sum  Inputs=-+
  Sum6 : Sum  Inputs=--+
  Sum7 : Sum  Inputs=---
  Eq1 : Outport
  Ed1 : Outport  Port=2
  Phi_1d : Outport  Port=3
  Phi_2q : Outport  Port=4
  wires:
  Efd/1 -> [Efd]
  Iq/1 -> [Iq]
  Id/1 -> [Id]
  Integrator3/1 -> Phi_2q/1, [Phi_2q]
  Sum7/1 -> Gain11/1
  [Ed1] -> Sum7/3
  [Phi_2q] -> Sum7/2
  Gain10/1 -> Sum7/1
  [Iq] -> Gain10/1
  Integrator2/1 -> Phi_1d/1, [Phi_1d]
  Sum6/1 -> Gain9/1
  [Eq1] -> Sum6/3
  [Phi_1d] -> Sum6/2
  Gain8/1 -> Sum6/1
  [Id] -> Gain8/1
  Sum5/1 -> Gain7/1
  Gain6/1 -> Sum5/2
  [Ed1] -> Sum5/1
  Sum4/1 -> Gain6/1
  Gain5/1 -> Sum4/2
  [Iq] -> Sum4/1
  Sum3/1 -> Gain5/1
  [Ed1] -> Sum3/3
  [Phi_2q] -> Sum3/2
  Gain4/1 -> Sum3/1
  [Iq] -> Gain4/1
  Integrator1/1 -> [Ed1], Ed1/1
  Sum2/1 -> Gain3/1
  [Efd] -> Sum2/3
  Gain2/1 -> Sum2/2
  [Eq1] -> Sum2/1
  Sum1/1 -> Gain2/1
  Gain1/1 -> Sum1/2
  [Id] -> Sum1/1
  Sum/1 -> Gain1/1
  [Eq1] -> Sum/3
  [Id] -> Gain/1
  Integrator/1 -> [Eq1], Eq1/1
  Gain/1 -> Sum/1
  [Phi_1d] -> Sum/2
  Temp/1 -> [R_temp_delta]
  [R_temp_delta] -> Product3/1
  Gain9/1 -> Product3/2
  Product3/1 -> Integrator2/1
  [R_temp_delta] -> Product1/1
  Gain11/1 -> Product1/2
  Product1/1 -> Integrator3/1
  [R_temp_delta] -> Product2/1
  Gain3/1 -> Product2/2
  Product2/1 -> Integrator/1
  [R_temp_delta] -> Product4/1
  Gain7/1 -> Product4/2
  Product4/1 -> Integrator1/1

== system Boeing787_OldMission_ElectricalThermalHydraulicFuelECS/Electrical/Generation Unit Sync-Sync1/Generator/Electromagnetic Torque Output Power ==
  note: Torque from Damper Windings
  note: Torque from Field Winding
  Id : Inport
  Iq : Inport  Port=2
  Eq1 : Inport  Port=3
  Ed1 : Inport  Port=4
  Phi_1d : Inport  Port=5
  Phi_2q : Inport  Port=6
  Gain : Gain  Gain=(Xd2 - Xls)/(Xd1 - Xls)
  Gain1 : Gain  Gain=(Xq2 - Xls)/(Xq1 - Xls)
  Gain2 : Gain  Gain=(Xd1 - Xd2)/(Xd1-Xls)
  Gain3 : Gain  Gain=(Xq1 - Xq2)/(Xq1-Xls)
  Gain4 : Gain  Gain=(Xq2 - Xd2)
  Product{,1..4} (5 alike) : Product  RndMeth=Zero
  Sum : Sum
  Sum1 : Sum  Inputs=+-+
  Sum2 : Sum
  TE : Outport
  wires:
  Sum2/1 -> TE/1
  Sum1/1 -> Sum2/2
  Sum/1 -> Sum2/1
  Gain1/1 -> Sum/2
  Gain/1 -> Sum/1
  Gain4/1 -> Sum1/3
  Gain2/1 -> Sum1/1
  Gain3/1 -> Sum1/2
  Product4/1 -> Gain4/1
  [Iq] -> Product4/2
  [Id] -> Product4/1
  Product3/1 -> Gain3/1
  [Phi_2q] -> Product3/2
  [Id] -> Product3/1
  Product2/1 -> Gain2/1
  [Phi_1d] -> Product2/2
  [Iq] -> Product2/1
  Product1/1 -> Gain1/1
  [Id] -> Product1/2
  [Ed1] -> Product1/1
  Product/1 -> Gain/1
  [Iq] -> Product/2
  [Eq1] -> Product/1
  Iq/1 -> [Iq]
  Phi_2q/1 -> [Phi_2q]
  Phi_1d/1 -> [Phi_1d]
  Ed1/1 -> [Ed1]
  Eq1/1 -> [Eq1]
  Id/1 -> [Id]

== system Boeing787_OldMission_ElectricalThermalHydraulicFuelECS/Electrical/Generation Unit Sync-Sync1/Generator/Generator Power Loss ==
  Ed : Inport
  Eq : Inport  Port=2
  Id : Inport  Port=3
  Iq : Inport  Port=4
  Te : Inport  Port=5
  w/ws : Inport  Port=6
  Bus Creator : BusCreator  Inputs=6
  Gain1 : Gain  Gain=SB
  Gain2 : Gain  Gain=SB
  Gain3 : Gain  Gain=SB
  Product : Product  RndMeth=Zero
  Product1 : Product  RndMeth=Zero
  Product2 : Product  RndMeth=Zero
  Sum1 : Sum  Inputs=-+
  Sum2 : Sum
  PE : Outport
  PM : Outport  Port=2
  PLOSS : Outport  Port=3
  m : Outport  Port=4
  wires:
  Gain3/1 -> PM/1
  Gain1/1 -> PE/1
  Gain2/1 -> PLOSS/1
  Bus Creator/1 -> m/1
  [nu] -> Bus Creator/6  "nu"
  [Te] -> Bus Creator/5  "Te"
  [Iq] -> Bus Creator/4  "Iq"
  [Eq] -> Bus Creator/3  "Vq"
  [Id] -> Bus Creator/2  "Id"
  [Ed] -> Bus Creator/1  "Vd"
  Sum1/1 -> Gain2/1
  Product2/1 -> Gain3/1, Sum1/2
  Sum2/1 -> Gain1/1, Sum1/1
  Product1/1 -> Sum2/2
  Product/1 -> Sum2/1
  [nu] -> Product2/2
  [Te] -> Product2/1
  [Iq] -> Product1/2
  [Eq] -> Product1/1
  [Id] -> Product/2
  [Ed] -> Product/1
  w/ws/1 -> [nu]
  Te/1 -> [Te]
  Iq/1 -> [Iq]
  Id/1 -> [Id]
  Eq/1 -> [Eq]
  Ed/1 -> [Ed]

== system Boeing787_OldMission_ElectricalThermalHydraulicFuelECS/Electrical/Generation Unit Sync-Sync1/Generator/Stator Voltage ==
  Id : Inport
  Iq : Inport  Port=2
  Eq1 : Inport  Port=3
  Ed1 : Inport  Port=4
  Phi_1d : Inport  Port=5
  Phi_2q : Inport  Port=6
  w/ws : Inport  Port=7
  Temp : Inport  Port=8
  Gain : Gain  Gain=(Xq2 - Xls)/(Xq1 - Xls)
  Gain1 : Gain  Gain=(Xq1 - Xq2)/(Xq1 - Xls)
  Gain2 : Gain  Gain=(Xq2 - Xd2)
  Gain3 : Gain  Gain=(Xd2 - Xls)/(Xd1 - Xls)
  Gain4 : Gain  Gain=(Xd1 - Xd2)/(Xd1 - Xls)
  Gain5 : Gain  Gain=Rs
  Gain6 : Gain  Gain=Xd2
  Gain7 : Gain  Gain=Rs
  Gain8 : Gain  Gain=Xd2
  Product{,1..3,5} (5 alike) : Product  RndMeth=Zero
  Product4 : Product
  Sum : Sum
  Sum1 : Sum  Inputs=+-+
  Sum2 : Sum  Inputs=--+
  Sum3 : Sum  Inputs=-++
  Ed : Outport
  Eq : Outport  Port=2
  wires:
  Gain7/1 -> Sum2/2
  Product3/1 -> Sum2/1
  Sum2/1 -> Eq/1  "Vq"
  Sum3/1 -> Ed/1  "Vd"
  Product2/1 -> Sum3/3
  Product1/1 -> Sum3/2
  Gain8/1 -> Product3/1
  Gain6/1 -> Product2/2
  Id/1 -> Gain8/1, Gain5/1
  Product/1 -> Sum2/3
  w/ws/1 -> Product2/1, Product3/2, Product/2, Product1/2
  Sum1/1 -> Product1/1
  Sum/1 -> Product/1
  Gain1/1 -> Sum1/2
  Gain/1 -> Sum1/1
  Gain3/1 -> Sum/1
  Gain4/1 -> Sum/2
  Phi_1d/1 -> Gain4/1
  Eq1/1 -> Gain3/1
  Phi_2q/1 -> Gain1/1
  Ed1/1 -> Gain/1
  Gain2/1 -> Sum1/3
  Temp/1 -> Product5/1, Product4/2
  Gain5/1 -> Product4/1
  Product4/1 -> Sum3/1
  Product5/1 -> Gain7/1
  Iq/1 -> Gain2/1, Product5/2, Gain6/1

== system Boeing787_OldMission_ElectricalThermalHydraulicFuelECS/Electrical/Generation Unit Sync-Sync2/Generator/Dynamics ==
  Id : Inport
  Iq : Inport  Port=2
  Efd : Inport  Port=3
  Temp : Inport  Port=4
  Gain : Gain  Gain=Xd1 - Xls
  Gain1 : Gain  Gain=(Xd1 - Xd2)/(Xd1-Xls)^2
  Gain10 : Gain  Gain=Xq1 - Xls
  Gain11 : Gain  Gain=1/Tqo2
  Gain2 : Gain  Gain=Xd - Xd1
  Gain3 : Gain  Gain=1/Tdo1
  Gain4 : Gain  Gain=Xq1 - Xls
  Gain5 : Gain  Gain=(Xq1 - Xq2)/(Xq1 - Xls)^2
  Gain6 : Gain  Gain=Xq - Xq1
  Gain7 : Gain  Gain=1/Tqo1
  Gain8 : Gain  Gain=Xd1 - Xls
  Gain9 : Gain  Gain=1/Tdo2
  Integrator{,1..3} (4 alike) : Integrator
  Product{1..4} (4 alike) : Product
  Sum : Sum  Inputs=++-
  Sum1 : Sum  Inputs=+-
  Sum2 : Sum  Inputs=--+
  Sum3 : Sum  Inputs=+++
  Sum4 : Sum  Inputs=+-
  Sum5 : Sum  Inputs=-+
  Sum6 : Sum  Inputs=--+
  Sum7 : Sum  Inputs=---
  Eq1 : Outport
  Ed1 : Outport  Port=2
  Phi_1d : Outport  Port=3
  Phi_2q : Outport  Port=4
  wires:
  Efd/1 -> [Efd]
  Iq/1 -> [Iq]
  Id/1 -> [Id]
  Integrator3/1 -> Phi_2q/1, [Phi_2q]
  Sum7/1 -> Gain11/1
  [Ed1] -> Sum7/3
  [Phi_2q] -> Sum7/2
  Gain10/1 -> Sum7/1
  [Iq] -> Gain10/1
  Integrator2/1 -> Phi_1d/1, [Phi_1d]
  Sum6/1 -> Gain9/1
  [Eq1] -> Sum6/3
  [Phi_1d] -> Sum6/2
  Gain8/1 -> Sum6/1
  [Id] -> Gain8/1
  Sum5/1 -> Gain7/1
  Gain6/1 -> Sum5/2
  [Ed1] -> Sum5/1
  Sum4/1 -> Gain6/1
  Gain5/1 -> Sum4/2
  [Iq] -> Sum4/1
  Sum3/1 -> Gain5/1
  [Ed1] -> Sum3/3
  [Phi_2q] -> Sum3/2
  Gain4/1 -> Sum3/1
  [Iq] -> Gain4/1
  Integrator1/1 -> [Ed1], Ed1/1
  Sum2/1 -> Gain3/1
  [Efd] -> Sum2/3
  Gain2/1 -> Sum2/2
  [Eq1] -> Sum2/1
  Sum1/1 -> Gain2/1
  Gain1/1 -> Sum1/2
  [Id] -> Sum1/1
  Sum/1 -> Gain1/1
  [Eq1] -> Sum/3
  [Id] -> Gain/1
  Integrator/1 -> [Eq1], Eq1/1
  Gain/1 -> Sum/1
  [Phi_1d] -> Sum/2
  Temp/1 -> [R_temp_delta]
  [R_temp_delta] -> Product3/1
  Gain9/1 -> Product3/2
  Product3/1 -> Integrator2/1
  [R_temp_delta] -> Product1/1
  Gain11/1 -> Product1/2
  Product1/1 -> Integrator3/1
  [R_temp_delta] -> Product2/1
  Gain3/1 -> Product2/2
  Product2/1 -> Integrator/1
  [R_temp_delta] -> Product4/1
  Gain7/1 -> Product4/2
  Product4/1 -> Integrator1/1
